simulink model "Exercise_4"  (R2020b)
settings: Solver=VariableStepAuto  StartTime=0.0  StopTime=0.1  RelTol=1e-3
libraries: fl_lib x12, nesl_utility x3, powerlib_meascontrol x1
settings Model: Creator=zaliyazici  LastModifiedBy=zaliyazici

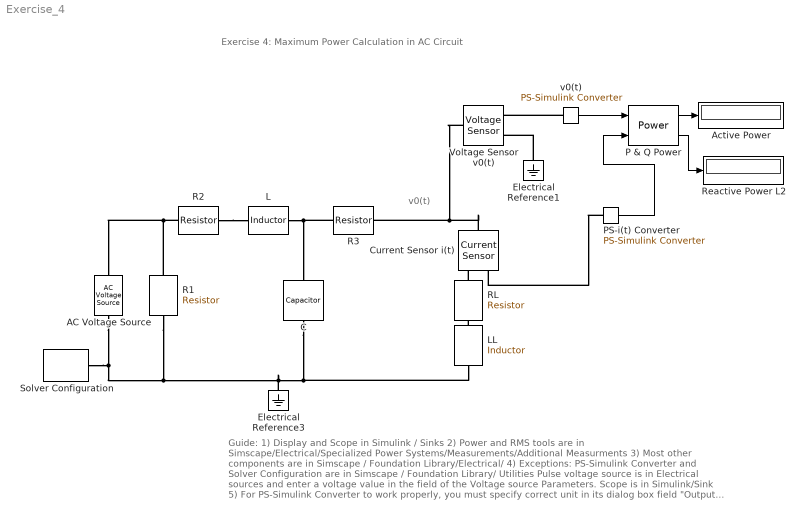
== system Exercise_4 ==
  note: Exercise 4: Maximum Power Calculation in AC Circuit
  note: v0(t)
  note: Guide:
      | 1) Display and Scope in Simulink / Sinks
      | 2) Power and RMS tools are in Simscape/Electrical/Specialized Power Systems/Measurements/Additional Measurments
      | 3) Most other components are in Simscape / Foundation Library/Electrical/
      | 4) Exceptions: PS-Simulink Converter and Solver Configuration are in Simscape / Foundation Library/ Utilities
      | Pulse voltage source is in Electrical sources and enter a voltage value in the field of the Voltage source Parameters.
      | Scope is in Simulink/Sink
      | 5) For PS-Simulink Converter to work properly, you must specify correct unit in its dialog box field "Output Signal Unit".
      | E.g. The unit must be A for Current sensor and V for Voltage sensor
      | 6) Solver Configuration f(x) = 0 is needed for setting info for simulation.
      | 7) To create "Annotation", double-click a location on project page and select "Create annotation" from the prompt. Then, type any text you want to clarify your circuit. E.g. "Display for Voltage".
      | 8) To understand how to use a component, right-click on the component and select "Help".
      | Measurement: Active and Reactive Powers
  AC Voltage Source : fl_lib/Electrical/Electrical Sources/AC Voltage Source  amp=160 V  shift=90 deg  frequency=60 Hz  omega=0 rad/s
      settings: AttributesFormatString=|
      | %<amp> %<amp_unit>
      | %<frequency> %<frequency_unit>
      | %<shift> %<shift_unit>
  "Active Power " : Display
  C : fl_lib/Electrical/Electrical Elements/Capacitor  c=10 uF  r=1e-6 Ohm  g=0 1/Ohm  i_specify=off  i_priority=None  i=0 A  i_nominal_specify=off  i_nominal_unit=A  i_nominal_value=1  v_specify=off  v_priority=None  v=0 V  v_nominal_specify=off  v_nominal_unit=V  v_nominal_value=1  vc_specify=off  vc_priority=High  vc=0 V  vc_nominal_specify=off  vc_nominal_unit=V  vc_nominal_value=1
      settings: AttributesFormatString=%<c> %<c_unit>
  Current Sensor i(t) : fl_lib/Electrical/Electrical Sensors/Current Sensor
  Electrical Reference1 : fl_lib/Electrical/Electrical Elements/Electrical Reference
  Electrical Reference3 : fl_lib/Electrical/Electrical Elements/Electrical Reference
  L : fl_lib/Electrical/Electrical Elements/Inductor  l=100 mH  r=0 Ohm  g=1e-9 1/Ohm  i_specify=off  i_priority=None  i=0 A  i_nominal_specify=off  i_nominal_unit=A  i_nominal_value=1  v_specify=off  v_priority=None  v=0 V  v_nominal_specify=off  v_nominal_unit=V  v_nominal_value=1  i_L_specify=off  i_L_priority=High  i_L=0 A  i_L_nominal_specify=off  i_L_nominal_unit=A  i_L_nominal_value=1
      settings: AttributesFormatString=%<l> %<l_unit>
  LL : fl_lib/Electrical/Electrical Elements/Inductor  l=1000 mH  r=0 Ohm  g=1e-9 1/Ohm  i_specify=off  i_priority=None  i=0 A  i_nominal_specify=off  i_nominal_unit=A  i_nominal_value=1  v_specify=off  v_priority=None  v=0 V  v_nominal_specify=off  v_nominal_unit=V  v_nominal_value=1  i_L_specify=off  i_L_priority=High  i_L=0 A  i_L_nominal_specify=off  i_L_nominal_unit=A  i_L_nominal_value=1
      settings: AttributesFormatString=%<l> %<l_unit>
  P & Q Power : powerlib_meascontrol/Measurements/Power  Freq=60  Vinit=[1, 0]  Iinit=[1, 0]  Ts=0
  PS-i(t) Converter : nesl_utility/PS-Simulink Converter  PhysicalDomain=network_engine_domain  SubClassName=ps_output  LeftPortType=input  RightPortType=output  PseudoPeriodic=off  Frequencies=[]  Unit=A  AffineConversion=off
  R1 : fl_lib/Electrical/Electrical Elements/Resistor  R=500 Ohm  i_specify=off  i_priority=None  i=0 A  i_nominal_specify=off  i_nominal_unit=A  i_nominal_value=1  v_specify=off  v_priority=None  v=0 V  v_nominal_specify=off  v_nominal_unit=V  v_nominal_value=1
      settings: AttributesFormatString=%<R> %<R_unit>  LogSimulationData=on
  R2 : fl_lib/Electrical/Electrical Elements/Resistor  R=250 Ohm  i_specify=off  i_priority=None  i=0 A  i_nominal_specify=off  i_nominal_unit=A  i_nominal_value=1  v_specify=off  v_priority=None  v=0 V  v_nominal_specify=off  v_nominal_unit=V  v_nominal_value=1
      settings: AttributesFormatString=%<R> %<R_unit>  LogSimulationData=on
  R3 : fl_lib/Electrical/Electrical Elements/Resistor  R=400 Ohm  i_specify=off  i_priority=None  i=0 A  i_nominal_specify=off  i_nominal_unit=A  i_nominal_value=1  v_specify=off  v_priority=None  v=0 V  v_nominal_specify=off  v_nominal_unit=V  v_nominal_value=1
      settings: AttributesFormatString=%<R> %<R_unit>  LogSimulationData=on
  RL : fl_lib/Electrical/Electrical Elements/Resistor  R=614 Ohm  i_specify=off  i_priority=None  i=0 A  i_nominal_specify=off  i_nominal_unit=A  i_nominal_value=1  v_specify=off  v_priority=None  v=0 V  v_nominal_specify=off  v_nominal_unit=V  v_nominal_value=1
      settings: LogSimulationData=on
  Reactive Power L2 : Display
  Solver Configuration : nesl_utility/Solver Configuration  PhysicalDomain=network_engine_domain  SubClassName=solver  LeftPortType=input  RightPortType=generic  Tones=[]  Harmonics=[]  SimulateNoise=off  Profile=off  UseLocalSampling=off  EnableSwitchedLinearOptims=on  FrequencyDomain=off  UseCCode=off  RelTol=0.001  AbsTol=1e-06  MinStep=1e-09  ToWorkspace=off  RevertToSquareIcSolve=off  NumHomotopyIterations=100  PhasorMode=off  PhasorModeNumHarmonics=1  DoDC=off  ResidualTolerance=1e-09  UseLocalSolver=off  LocalSolverChoice=NE_BACKWARD_EULER_ADVANCER  LocalSolverSampleTime=0.001  DoFixedCost=off  MaxNonlinIter=3  MaxModeIter=2  ComputeImpulses=off  ImpulseIterations=2  LinearAlgebra=auto  EquationFormulation=NE_TIME_EF  DelaysMemoryBudget=1024  AutomaticFiltering=on  FilteringTimeConstant=0.001  PartitionStorageMethod=AS_NEEDED  PartitionMemoryBudget=1024  PartitionMethod=ROBUST
  Voltage Sensor v0(t) : fl_lib/Electrical/Electrical Sensors/Voltage Sensor
  v0(t) : nesl_utility/PS-Simulink Converter  PhysicalDomain=network_engine_domain  SubClassName=ps_output  LeftPortType=input  RightPortType=output  PseudoPeriodic=off  Frequencies=[]  Unit=V  AffineConversion=off
  wires:
  P & Q Power/2 -> Reactive Power L2/1
  v0(t)/1 -> P & Q Power/1
  P & Q Power/1 -> "Active Power "/1
  PS-i(t) Converter/1 -> P & Q Power/2
  connections:
  R2/LConn1 -- R1/RConn1 -- AC Voltage Source/LConn1
  Electrical Reference1/LConn1 -- Voltage Sensor v0(t)/RConn2
  RL/LConn1 -- Current Sensor i(t)/RConn2
  v0(t)/LConn1 -- Voltage Sensor v0(t)/RConn1
  PS-i(t) Converter/LConn1 -- Current Sensor i(t)/RConn1
  R2/RConn1 -- L/LConn1
  AC Voltage Source/RConn1 -- Solver Configuration/RConn1 -- R1/LConn1 -- Electrical Reference3/LConn1 -- LL/RConn1 -- C/RConn1
  LL/LConn1 -- RL/RConn1
  L/RConn1 -- R3/LConn1 -- C/LConn1
  Current Sensor i(t)/LConn1 -- Voltage Sensor v0(t)/LConn1 -- R3/RConn1
